simulink model "scheme"  (R2022b)
settings: Solver=VariableStepAuto  StartTime=0.0  StopTime=10.0  RelTol=1e-3
libraries: slpidlib x1
settings Model: Creator=elife  LastModifiedBy=elife

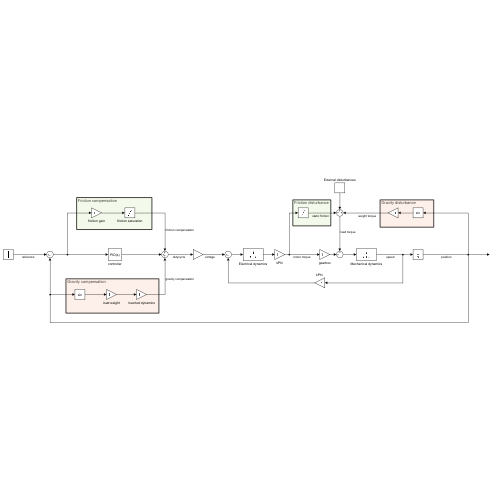
[thumbnail: Simulink's stored preview of the top-level diagram]
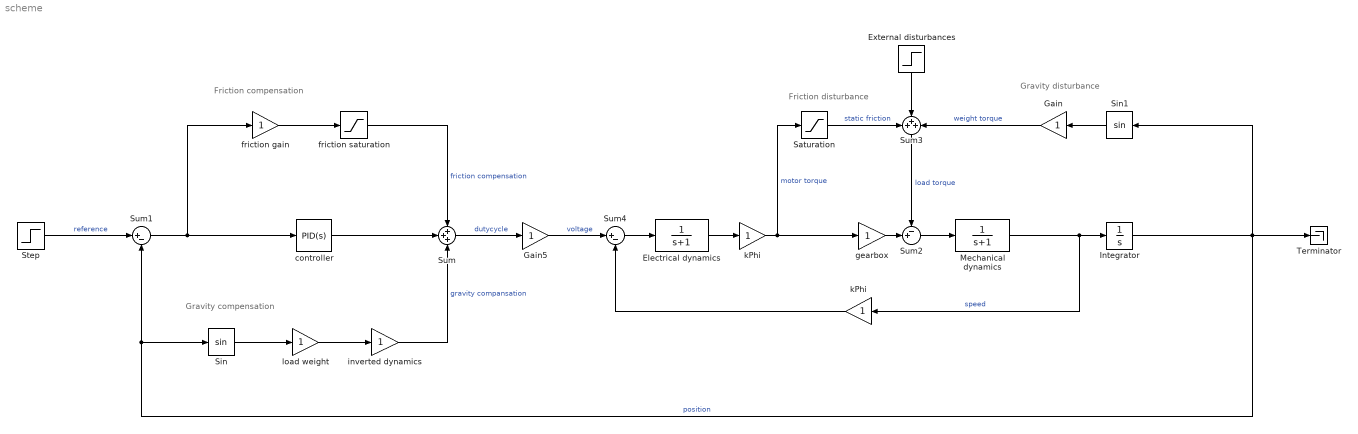
== system scheme ==
  note: Friction disturbance
  note: Gravity disturbance
  note: Friction compensation
  note: Gravity compensation
  Electrical dynamics : TransferFcn  Denominator=[1 1]
  External disturbances : Step  SampleTime=0
  Gain : Gain
  Gain5 : Gain
  Integrator : Integrator
  Mechanical dynamics : TransferFcn  Denominator=[1 1]
  Saturation : Saturate
  Sin : Trigonometry
  Sin1 : Trigonometry
  Step : Step  SampleTime=0
  Sum : Sum  Inputs=+++
  Sum1 : Sum  Inputs=|+-
  Sum2 : Sum  Inputs=-+|
  Sum3 : Sum  Inputs=+++
  Sum4 : Sum  Inputs=|+-
  Terminator : Terminator
  controller : slpidlib/PID Controller  Controller=PID  Form=Parallel  TimeDomain=Continuous-time  UseExternalTs=off  SampleTime=-1  IntegratorMethod=Forward Euler  FilterMethod=Forward Euler  ControllerParametersSource=internal  P=1  I=1  UseKiTs=off  D=0  N=100  UseFilter=on  TunerSelectOption=Transfer Function Based (PID Tuner App)  InitialConditionSource=internal  InitialConditionForIntegrator=0  InitialConditionForFilter=0  DifferentiatorICPrevScaledInput=0  ExternalReset=none  TrackingMode=off  Kt=1  LimitOutput=off  SatLimitsSource=internal  UpperSaturationLimit=inf  LowerSaturationLimit=-inf  LinearizeAsGain=on  AntiWindupMode=none  Kb=1  LimitIntegrator=off  UpperIntegratorSaturationLimit=inf  LowerIntegratorSaturationLimit=-inf  POutMin=[]  POutMax=[]  IOutMin=[]  IOutMax=[]  DOutMin=[]  DOutMax=[]  NOutMin=[]  NOutMax=[]  SumOutMin=[]  SumOutMax=[]  SaturationOutMin=[]  SaturationOutMax=[]  PParamMin=[]  PParamMax=[]  IParamMin=[]  IParamMax=[]  DParamMin=[]  DParamMax=[]  NParamMin=[]  NParamMax=[]  KbParamMin=[]  KbParamMax=[]  KtParamMin=[]  KtParamMax=[]  KbOutMin=[]  KbOutMax=[]  KtOutMin=[]  KtOutMax=[]  IntegratorOutMin=[]  IntegratorOutMax=[]  FilterOutMin=[]  FilterOutMax=[]  SumI1OutMin=[]  SumI1OutMax=[]  SumI2OutMin=[]  SumI2OutMax=[]  SumI3OutMin=[]  SumI3OutMax=[]  SumI4OutMin=[]  SumI4OutMax=[]  SumDOutMin=[]  SumDOutMax=[]  DifferentiatorOutMin=[]  DifferentiatorOutMax=[]  FilterDiffOutCoefMin=[]  FilterDiffOutCoefMax=[]  ReciprocalOutMin=[]  ReciprocalOutMax=[]  SumDenOutMin=[]  SumDenOutMax=[]  SumNumOutMin=[]  SumNumOutMax=[]  DivideOutMin=[]  DivideOutMax=[]  UdiffTsProdOutMin=[]  UdiffTsProdOutMax=[]  NTsProdOutMin=[]  NTsProdOutMax=[]  UintegralTsProdOutMin=[]  UintegralTsProdOutMax=[]  UngainTsProdOutMin=[]  UngainTsProdOutMax=[]  ClampingZeroOutDataTypeStr=Inherit: Inherit via back propagation  ClampingZeroOutMin=[]  ClampingZeroOutMax=[]  FilterDenConstantOutDataTypeStr=Inherit: Inherit via back propagation  FilterDenConstantOutMin=[]  FilterDenConstantOutMax=[]  PCopyOutDataTypeStr=Inherit: Inherit via back propagation  PCopyOutMin=[]  PCopyOutMax=[]  NCopyOutDataTypeStr=Inherit: Inherit via back propagation  NCopyOutMin=[]  NCopyOutMax=[]  IntegratorContinuousStateAttributes=''  IntegratorStateMustResolveToSignalObject=off  IntegratorRTWStateStorageClass=Auto  FilterContinuousStateAttributes=''  FilterStateMustResolveToSignalObject=off  FilterRTWStateStorageClass=Auto  ParallelPVariant=InternalParameters  IdealPVariant=Disabled  IVariant=InternalParameters  DVariant=InternalParameters  IntegratorVariant=Continuous  SatVariant=Disabled  AWVariant=Passthrough  PCopyVariant=Disabled  TRVariant=Disabled  FdbkBlocksVariant=Forward  IdealPFdbkVariant=Disabled  SatFdbkVariant=Disabled  DerivativeFilterVariant=ContFilter  NVariant=InternalParameters  NCopyVariant=Disabled  FilterICVariant=InternalICsFilter  IntegratorICVariant=InternalICs  ExternalResetVariant=Disabled  TRSumVariant=Passthrough  SumFdbkVariant=Disabled  SumVariant=Sum_PID  TsampFilterVariant=InternalTs  TsampNgainVariant=Passthrough  TsampIntegralVariant=Passthrough  ExternalSaturationOutDataTypeStr=Inherit: Same as second input
  friction gain : Gain
  friction saturation : Saturate
  gearbox : Gain
  inverted dynamics : Gain
  kPhi : Gain
  "kPhi " : Gain
  load weight : Gain
  wires:
  Sin/1 -> load weight/1
  load weight/1 -> inverted dynamics/1
  inverted dynamics/1 -> Sum/3  "gravity compansation"
  controller/1 -> Sum/2
  Sum1/1 -> friction gain/1, controller/1
  friction gain/1 -> friction saturation/1
  friction saturation/1 -> Sum/1  "friction compensation"
  Sum/1 -> Gain5/1  "dutycycle"
  Step/1 -> Sum1/1  "reference"
  Electrical dynamics/1 -> kPhi/1
  Sum2/1 -> Mechanical dynamics/1
  Mechanical dynamics/1 -> "kPhi "/1, Integrator/1  "speed"
  Integrator/1 -> Sin1/1, Sum1/2, Sin/1, Terminator/1  "position"
  Sin1/1 -> Gain/1
  Sum3/1 -> Sum2/1  "load torque"
  Gain/1 -> Sum3/3  "weight torque"
  Saturation/1 -> Sum3/1  "static friction"
  External disturbances/1 -> Sum3/2
  kPhi/1 -> gearbox/1, Saturation/1  "motor torque"
  Sum4/1 -> Electrical dynamics/1
  Gain5/1 -> Sum4/1  "voltage"
  "kPhi "/1 -> Sum4/2
  gearbox/1 -> Sum2/2
